simulink model "Aktuator_Steuer"  (R2019b)
settings: Solver=FixedStepAuto  StartTime=0.0  StopTime=1  FixedStep=0.00001  RelTol=1e-3
values from neighbouring files (symbols this model uses):
  Axialkraft = 3000    [Init_Aktuator_Steuer.m]
  Drehzahlkonstante = 1070    [Init_Aktuator.m]    (also in Init_Aktuator_Klapp.m = 569; Init_Aktuator_Steuer.m)
  Effizienz = 0.9    [Init_Aktuator_Steuer.m]
  Hebel1 = 208    [Init_Aktuator_Steuer.m]
  Hebel2 = 265    [Init_Aktuator_Steuer.m]
  I_Konstante = 20    [Init_Aktuator.m]    (also in Init_Aktuator_Steuer.m)
  Moment_aero = 255.25    [Init_Aktuator.m]    (also in Init_Aktuator_Steuer.m)
  Momentenkonstante = 8.95/1000    (= 0.00895)    [Init_Aktuator.m]    (also in Init_Aktuator_Klapp.m = 0.0168; Init_Aktuator_Steuer.m)
  P_Konstante = 4    [Init_Aktuator.m]    (also in Init_Aktuator_Steuer.m)
  Radialkraft = 6000    [Init_Aktuator_Steuer.m]
  Reibungsbeiwert = 0.0018    [Init_Aktuator_Steuer.m]
  Sollwert0 = 20    [Init_Aktuator.m]    (also in Init_Aktuator_Steuer.m)
  Sollwert1 = -20    [Init_Aktuator.m]    (also in Init_Aktuator_Steuer.m)
  Sollwert2 = 0    [Init_Aktuator.m]    (also in Init_Aktuator_Steuer.m)
  Spannung = 12    [Init_Aktuator_Klapp.m]
  Spannung_max = Nennspannung * 2    (= 24)    [Init_Aktuator.m]    (also in Init_Aktuator_Steuer.m = 18)
  Startauslenkung = 0/180*pi    (= 0)    [Init_Aktuator.m]    (also in Init_Aktuator_Steuer.m)
  Steigung = 27.1*1000    (= 27100)    [Init_Aktuator.m]    (also in Init_Aktuator_Klapp.m = 0.002; Init_Aktuator_Steuer.m)
  t1 = Periodendauer/4    (= 0.1825)    [Init_Aktuator.m]    (also in Init_Aktuator_Steuer.m)
  t2 = Periodendauer * 3/4    (= 0.5475)    [Init_Aktuator.m]    (also in Init_Aktuator_Steuer.m)
  Traegheitsmoment_gesamt = Traegheitsmoment_GF + Traegheitsmoment_Motor/Uebersetzung + Traegheitsmoment_Getriebe + Traegheitsmoment_Welle + Masse_Hubakuatorik * Abstand_Hubaktuatorik^2    (= 0.06555501325)    [Init_Aktuator_Steuer.m]
  Uebersetzung = 200    [Init_Aktuator.m]    (also in Init_Aktuator_Klapp.m = 3.7; Init_Aktuator_Steuer.m)
libraries: simulink x2
settings Model: Creator=Neu1  LastModifiedBy=Neu1

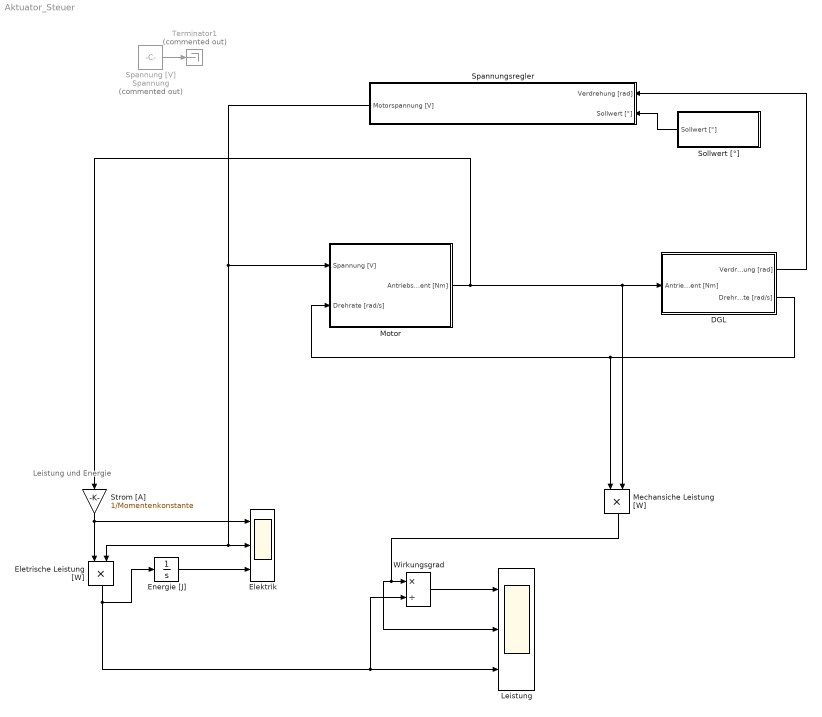
== system Aktuator_Steuer ==
  note: Leistung und Energie
  DGL : Subsystem
  "Elektrik " : Scope  NumInputPorts=3
  Eletrische Leistung [W] : Product
  Energie [J] : Integrator
  Leistung : Scope  NumInputPorts=3
  "Mechansiche Leistung [W] " : Product
  Motor : Subsystem
  Sollwert [°] : Subsystem
  Spannung [V] : Constant  Commented=on  Value=Spannung
  Spannungsregler : Subsystem
  Strom [A] : Gain  Gain=1/Momentenkonstante
  Terminator1 : Terminator  Commented=on
  Wirkungsgrad : Product  Inputs=*/
  wires:
  "Mechansiche Leistung [W] "/1 -> Leistung/2, Wirkungsgrad/1
  Strom [A]/1 -> Eletrische Leistung [W]/1, "Elektrik "/1
  Eletrische Leistung [W]/1 -> Energie [J]/1, Leistung/3, Wirkungsgrad/2
  Wirkungsgrad/1 -> Leistung/1
  Energie [J]/1 -> "Elektrik "/3
  Spannung [V]/1 -> Terminator1/1
  Motor/1(Antriebsmoment [Nm]) -> Strom [A]/1, DGL/1(Antriebsmoment [Nm]), "Mechansiche Leistung [W] "/2
  Spannungsregler/1(Motorspannung [V]) -> Motor/1(Spannung [V]), "Elektrik "/2, Eletrische Leistung [W]/2
  DGL/1(Verdrehung [rad]) -> Spannungsregler/1(Verdrehung [rad])
  DGL/2(Drehrate [rad/s]) -> Motor/2(Drehrate [rad/s]), "Mechansiche Leistung [W] "/1
  Sollwert [°]/1(Sollwert [°]) -> Spannungsregler/2(Sollwert [°])

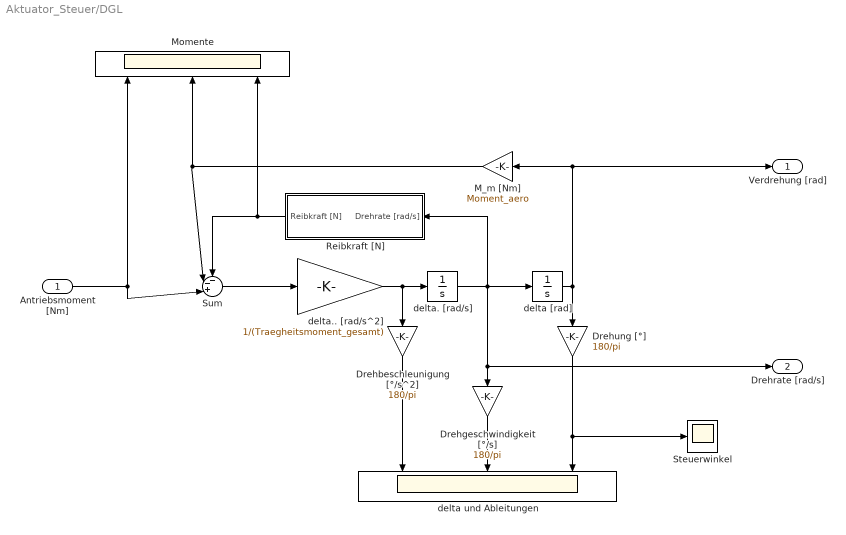
== system Aktuator_Steuer/DGL ==
  Antriebsmoment [Nm] : Inport
  Drehbeschleunigung [°/s^2] : Gain  Gain=180/pi
  Drehgeschwindigkeit [°/s] : Gain  Gain=180/pi
  Drehung [°] : Gain  Gain=180/pi
  M_m [Nm] : Gain  Gain=Moment_aero
  Momente : Scope  NumInputPorts=3
  Reibkraft [N] : Subsystem
  Steuerwinkel : Scope
  Sum : Sum  Inputs=--+|
  delta [rad] : Integrator  InitialCondition=Startauslenkung  WrapState=on
  delta und Ableitungen : Scope  NumInputPorts=3
  delta. [rad/s] : Integrator
  delta.. [rad/s^2] : Gain  Gain=1/(Traegheitsmoment_gesamt)
  Verdrehung [rad] : Outport
  Drehrate [rad/s] : Outport  Port=2
  wires:
  Sum/1 -> delta.. [rad/s^2]/1
  delta [rad]/1 -> Drehung [°]/1, M_m [Nm]/1, Verdrehung [rad]/1
  Drehung [°]/1 -> delta und Ableitungen/3, Steuerwinkel/1
  delta.. [rad/s^2]/1 -> delta. [rad/s]/1, Drehbeschleunigung [°/s^2]/1
  Drehgeschwindigkeit [°/s]/1 -> delta und Ableitungen/2
  Drehbeschleunigung [°/s^2]/1 -> delta und Ableitungen/1
  delta. [rad/s]/1 -> Reibkraft [N]/1("Drehrate [rad/s] "), Drehrate [rad/s]/1, Drehgeschwindigkeit [°/s]/1, delta [rad]/1
  Antriebsmoment [Nm]/1 -> Sum/3, Momente/1
  M_m [Nm]/1 -> Sum/2, Momente/2
  Reibkraft [N]/1(Reibkraft [N]) -> Sum/1, Momente/3

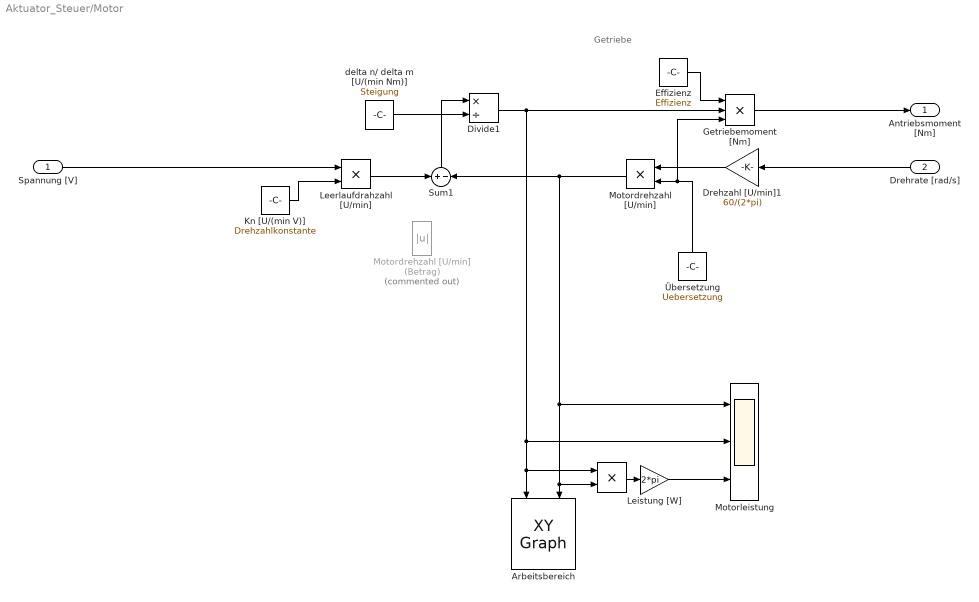
== system Aktuator_Steuer/Motor ==
  note: Getriebe
  Spannung [V] : Inport
  Drehrate [rad/s] : Inport  Port=2
  " " : Product
  "Arbeitsbereich " : simulink/Sinks/XY Graph  xmin=-1  xmax=1  ymin=-25000  ymax=30000  st=0.1
  Divide1 : Product  Inputs=*/
  Drehzahl [U/min]1 : Gain  Gain=60/(2*pi)
  Effizienz : Constant  Value=Effizienz
  Getriebemoment [Nm] : Product  Inputs=3
  Kn [U/(min V)] : Constant  Value=Drehzahlkonstante
  Leerlaufdrahzahl [U/min] : Product
  Leistung [W] : Gain  Gain=2*pi
  "Motordrehzahl [U/min] " : Product  Inputs=**
  Motordrehzahl [U/min] (Betrag) : Abs  Commented=on
  Motorleistung : Scope  NumInputPorts=3
  Sum1 : Sum  Inputs=+|-
  delta n/ delta m [U/(min Nm)] : Constant  Value=Steigung
  Übersetzung : Constant  Value=Uebersetzung
  Antriebsmoment [Nm] : Outport
  wires:
  delta n/ delta m [U/(min Nm)]/1 -> Divide1/2
  Sum1/1 -> Divide1/1
  Spannung [V]/1 -> Leerlaufdrahzahl [U/min]/1
  Leerlaufdrahzahl [U/min]/1 -> Sum1/1
  Kn [U/(min V)]/1 -> Leerlaufdrahzahl [U/min]/2
  Drehzahl [U/min]1/1 -> "Motordrehzahl [U/min] "/1
  Übersetzung/1 -> Getriebemoment [Nm]/3, "Motordrehzahl [U/min] "/2
  Getriebemoment [Nm]/1 -> Antriebsmoment [Nm]/1
  Effizienz/1 -> Getriebemoment [Nm]/1
  Drehrate [rad/s]/1 -> Drehzahl [U/min]1/1
  " "/1 -> Leistung [W]/1
  Divide1/1 -> Getriebemoment [Nm]/2, " "/1, "Arbeitsbereich "/1, Motorleistung/2
  "Motordrehzahl [U/min] "/1 -> Sum1/2, " "/2, "Arbeitsbereich "/2, Motorleistung/1
  Leistung [W]/1 -> Motorleistung/3

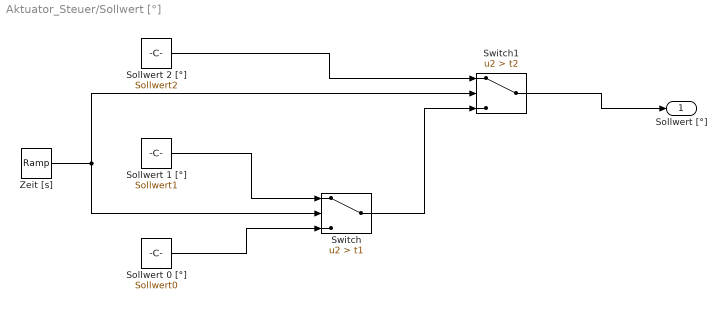
== system Aktuator_Steuer/Sollwert [°] ==
  Sollwert 0 [°] : Constant  Value=Sollwert0
  Sollwert 1 [°] : Constant  Value=Sollwert1
  Sollwert 2 [°] : Constant  Value=Sollwert2
  Switch : Switch  Criteria=u2 > Threshold  Threshold=t1
  Switch1 : Switch  Criteria=u2 > Threshold  Threshold=t2
  Zeit [s] : simulink/Sources/Ramp  slope=1  start=0  InitialOutput=0
  Sollwert [°] : Outport
  wires:
  Switch1/1 -> Sollwert [°]/1
  Zeit [s]/1 -> Switch/2, Switch1/2
  Switch/1 -> Switch1/3
  Sollwert 1 [°]/1 -> Switch/1
  Sollwert 0 [°]/1 -> Switch/3
  Sollwert 2 [°]/1 -> Switch1/1

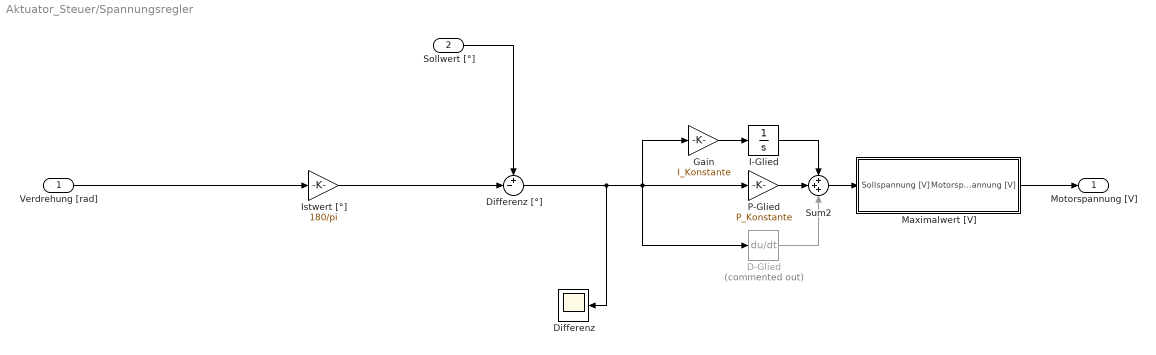
== system Aktuator_Steuer/Spannungsregler ==
  Verdrehung [rad] : Inport
  Sollwert [°] : Inport  Port=2
  D-Glied : Derivative  Commented=on  CoefficientInTFapproximation=D_Konstante
  Differenz : Scope
  Differenz [°] : Sum  Inputs=+-|
  Gain : Gain  Gain=I_Konstante
  I-Glied : Integrator
  Istwert [°] : Gain  Gain=180/pi
  Maximalwert [V] : Subsystem
  P-Glied : Gain  Gain=P_Konstante
  Sum2 : Sum  Inputs=+++
  Motorspannung [V] : Outport
  wires:
  Sum2/1 -> Maximalwert [V]/1("Sollspannung [V] ")
  Gain/1 -> I-Glied/1
  D-Glied/1 -> Sum2/3
  Differenz [°]/1 -> Gain/1, P-Glied/1, D-Glied/1, Differenz/1
  P-Glied/1 -> Sum2/2
  Sollwert [°]/1 -> Differenz [°]/1
  I-Glied/1 -> Sum2/1
  Istwert [°]/1 -> Differenz [°]/2
  Verdrehung [rad]/1 -> Istwert [°]/1
  Maximalwert [V]/1("Motorspannung [V] ") -> Motorspannung [V]/1

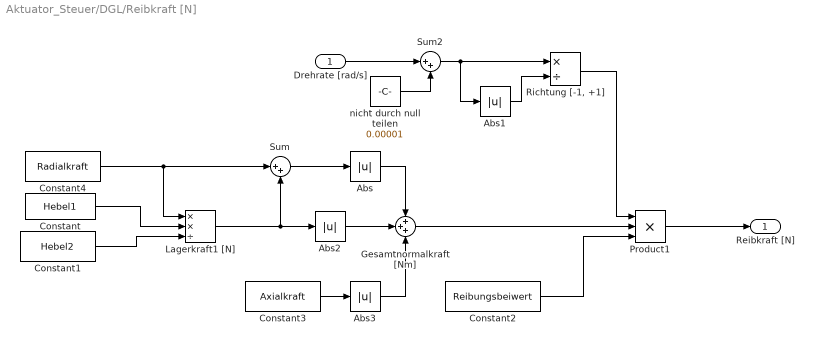
== system Aktuator_Steuer/DGL/Reibkraft [N] ==
  "Drehrate [rad/s] " : Inport
  Abs{,1..3} (4 alike) : Abs
  Constant : Constant  Value=Hebel1
  Constant1 : Constant  Value=Hebel2
  Constant2 : Constant  Value=Reibungsbeiwert
  Constant3 : Constant  Value=Axialkraft
  Constant4 : Constant  Value=Radialkraft
  Gesamtnormalkraft [Nm] : Sum  Inputs=+++
  Lagerkraft1 [N] : Product  Inputs=**/
  Product1 : Product  Inputs=3
  "Richtung [-1, +1]" : Product  Inputs=*/
  Sum : Sum  Inputs=|++
  Sum2 : Sum  Inputs=|++
  nicht durch null teilen : Constant  Value=0.00001
  Reibkraft [N] : Outport
  wires:
  Constant/1 -> Lagerkraft1 [N]/2
  Constant1/1 -> Lagerkraft1 [N]/3
  Constant4/1 -> Sum/1, Lagerkraft1 [N]/1
  Lagerkraft1 [N]/1 -> Abs2/1, Sum/2
  Sum/1 -> Abs/1
  Abs/1 -> Gesamtnormalkraft [Nm]/1
  Constant3/1 -> Abs3/1
  Abs1/1 -> "Richtung [-1, +1]"/2
  "Richtung [-1, +1]"/1 -> Product1/1
  Gesamtnormalkraft [Nm]/1 -> Product1/2
  Constant2/1 -> Product1/3
  Product1/1 -> Reibkraft [N]/1
  "Drehrate [rad/s] "/1 -> Sum2/1
  nicht durch null teilen/1 -> Sum2/2
  Sum2/1 -> "Richtung [-1, +1]"/1, Abs1/1
  Abs2/1 -> Gesamtnormalkraft [Nm]/2
  Abs3/1 -> Gesamtnormalkraft [Nm]/3

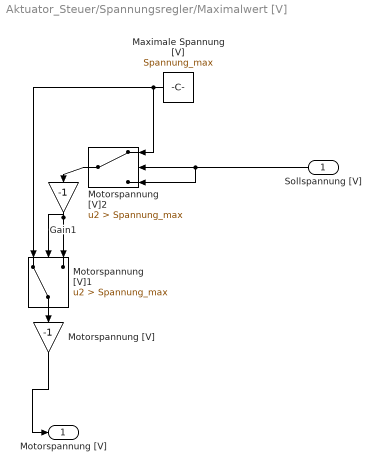
== system Aktuator_Steuer/Spannungsregler/Maximalwert [V] ==
  "Sollspannung [V] " : Inport
  Gain1 : Gain  Gain=-1
  Maximale Spannung [V] : Constant  Value=Spannung_max
  Motorspannung [V] : Gain  Gain=-1
  Motorspannung [V]1 : Switch  Criteria=u2 > Threshold  Threshold=Spannung_max
  Motorspannung [V]2 : Switch  Criteria=u2 > Threshold  Threshold=Spannung_max
  "Motorspannung [V] " : Outport
  wires:
  Motorspannung [V]2/1 -> Gain1/1
  Gain1/1 -> Motorspannung [V]1/2, Motorspannung [V]1/3
  "Sollspannung [V] "/1 -> Motorspannung [V]2/3, Motorspannung [V]2/2
  Maximale Spannung [V]/1 -> Motorspannung [V]1/1, Motorspannung [V]2/1
  Motorspannung [V]1/1 -> Motorspannung [V]/1
  Motorspannung [V]/1 -> "Motorspannung [V] "/1
